simulink model "Ejercicio_Teorica_Simulink_1_MK2"  (R2024a)
settings: Solver=VariableStepAuto  StartTime=0.0  StopTime=20.0  RelTol=1e-3
undefined symbols (not defined in the file or in its folder): C, mat_K, mat_K_ampliada, mat_Ki, sustitu_mat_lin_A, sustitu_mat_lin_B
settings Model: Creator=juanj  LastModifiedBy=juanj
settings RTWCC: GPUComputeCapability=3.5

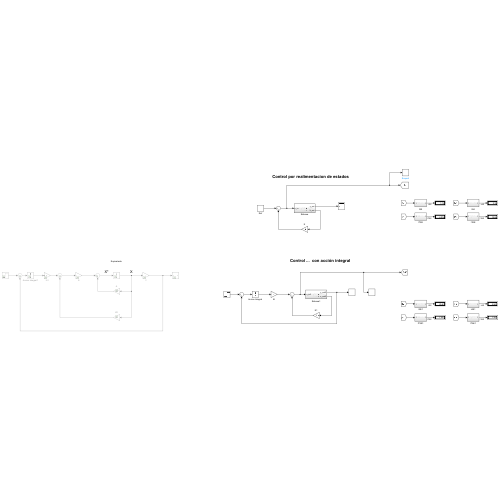
[thumbnail: Simulink's stored preview of the top-level diagram]
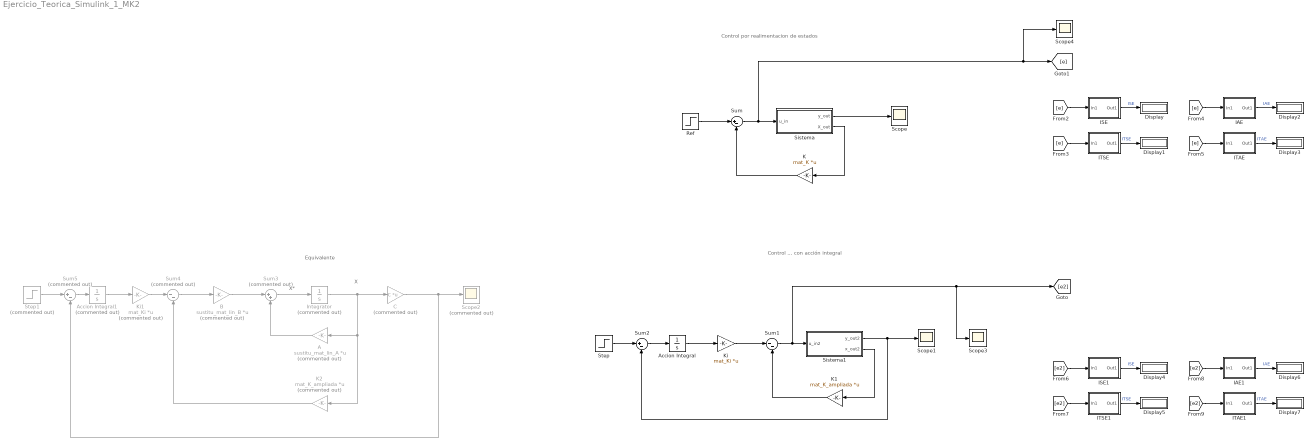
== system Ejercicio_Teorica_Simulink_1_MK2 ==
  note: Control ... con acción integral
  note: Equivalente
  note: X*
  note: X
  note: Control por realimentacion de estados
  A : Gain  Commented=on  Gain=sustitu_mat_lin_A  Multiplication=Matrix(K*u)
  Accion Integral : Integrator
  Accion Integral1 : Integrator  Commented=on
  B : Gain  Commented=on  Gain=sustitu_mat_lin_B  Multiplication=Matrix(K*u)
  C : Gain  Commented=on  Gain=C  Multiplication=Matrix(K*u)
  Display{,1..7} (8 alike) : Display
  IAE : Subsystem
  IAE1 : Subsystem
  ISE : Subsystem
  ISE1 : Subsystem
  ITAE : Subsystem
  ITAE1 : Subsystem
  ITSE : Subsystem
  ITSE1 : Subsystem
  Integrator : Integrator  Commented=on
  K : Gain  Gain=mat_K  Multiplication=Matrix(K*u)
  K1 : Gain  Gain=mat_K_ampliada  Multiplication=Matrix(K*u)
  K2 : Gain  Commented=on  Gain=mat_K_ampliada  Multiplication=Matrix(K*u)
  Ki : Gain  Gain=mat_Ki  Multiplication=Matrix(K*u)
  Ki1 : Gain  Commented=on  Gain=mat_Ki  Multiplication=Matrix(K*u)
  Ref : Step  Time=0  SampleTime=0
  Scope{,1,3..4} (4 alike) : Scope
  Scope2 : Scope  Commented=on
  Sistema : Subsystem
  Sistema1 : Subsystem
  Step : Step  Time=0  SampleTime=0
  Step1 : Step  Commented=on  Time=0  SampleTime=0
  Sum : Sum  Inputs=|+-
  Sum1 : Sum  Inputs=|--
  Sum2 : Sum  Inputs=|+-
  Sum3 : Sum  Commented=on  Inputs=|++
  Sum4 : Sum  Commented=on  Inputs=|--
  Sum5 : Sum  Commented=on  Inputs=|+-
  wires:
  Ref/1 -> Sum/1
  Sistema/1(y_out) -> Scope/1
  Sistema/2(X_out) -> K/1
  K/1 -> Sum/2
  Sistema1/1(y_out2) -> Scope1/1, Sum2/2
  Accion Integral/1 -> Ki/1
  Sum2/1 -> Accion Integral/1
  K1/1 -> Sum1/2
  Ki/1 -> Sum1/1
  Step/1 -> Sum2/1
  Sistema1/2(x_out2) -> K1/1
  Sum3/1 -> Integrator/1
  Sum4/1 -> B/1
  Integrator/1 -> K2/1, A/1, C/1
  A/1 -> Sum3/2
  B/1 -> Sum3/1
  K2/1 -> Sum4/2
  Ki1/1 -> Sum4/1
  Accion Integral1/1 -> Ki1/1
  Step1/1 -> Sum5/1
  Sum5/1 -> Accion Integral1/1
  C/1 -> Sum5/2, Scope2/1
  [e] -> ISE/1(In1)
  ISE/1(Out1) -> Display/1  "ISE"
  [e] -> ITAE/1(In1)
  ITSE/1(Out1) -> Display1/1  "ITSE"
  [e] -> ITSE/1(In1)
  ITAE/1(Out1) -> Display3/1  "ITAE"
  [e] -> IAE/1(In1)
  IAE/1(Out1) -> Display2/1  "IAE"
  [e2] -> ITAE1/1(In1)
  [e2] -> ISE1/1(In1)
  [e2] -> IAE1/1(In1)
  [e2] -> ITSE1/1(In1)
  ITAE1/1(Out1) -> Display7/1  "ITAE"
  IAE1/1(Out1) -> Display6/1  "IAE"
  ITSE1/1(Out1) -> Display5/1  "ITSE"
  ISE1/1(Out1) -> Display4/1  "ISE"
  Sum/1 -> Sistema/1(u_in), Scope4/1, [e]
  Sum1/1 -> [e2], Scope3/1, Sistema1/1(u_in2)

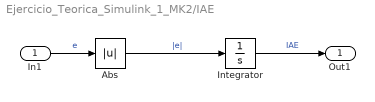
== system Ejercicio_Teorica_Simulink_1_MK2/IAE ==
  In1 : Inport
  Abs : Abs  SaturateOnIntegerOverflow=off
  Integrator : Integrator
  Out1 : Outport
  wires:
  Integrator/1 -> Out1/1  "IAE"
  In1/1 -> Abs/1  "e"
  Abs/1 -> Integrator/1  "|e|"

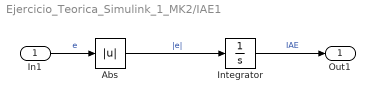
== system Ejercicio_Teorica_Simulink_1_MK2/IAE1 ==
  In1 : Inport
  Abs : Abs  SaturateOnIntegerOverflow=off
  Integrator : Integrator
  Out1 : Outport
  wires:
  Integrator/1 -> Out1/1  "IAE"
  In1/1 -> Abs/1  "e"
  Abs/1 -> Integrator/1  "|e|"

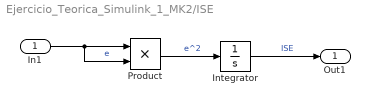
== system Ejercicio_Teorica_Simulink_1_MK2/ISE ==
  In1 : Inport
  Integrator : Integrator
  Product : Product
  Out1 : Outport
  wires:
  In1/1 -> Product/2, Product/1  "e"
  Product/1 -> Integrator/1  "e^2"
  Integrator/1 -> Out1/1  "ISE"

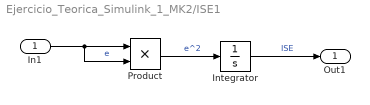
== system Ejercicio_Teorica_Simulink_1_MK2/ISE1 ==
  In1 : Inport
  Integrator : Integrator
  Product : Product
  Out1 : Outport
  wires:
  In1/1 -> Product/2, Product/1  "e"
  Product/1 -> Integrator/1  "e^2"
  Integrator/1 -> Out1/1  "ISE"

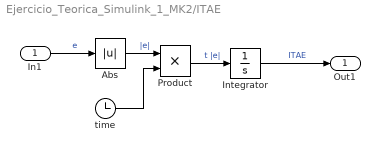
== system Ejercicio_Teorica_Simulink_1_MK2/ITAE ==
  In1 : Inport
  Abs : Abs  SaturateOnIntegerOverflow=off
  Integrator : Integrator
  Product : Product
  time : Clock
  Out1 : Outport
  wires:
  In1/1 -> Abs/1  "e"
  Integrator/1 -> Out1/1  "ITAE"
  time/1 -> Product/2
  Abs/1 -> Product/1  "|e|"
  Product/1 -> Integrator/1  "t |e|"

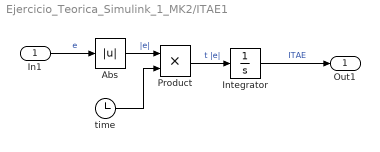
== system Ejercicio_Teorica_Simulink_1_MK2/ITAE1 ==
  In1 : Inport
  Abs : Abs  SaturateOnIntegerOverflow=off
  Integrator : Integrator
  Product : Product
  time : Clock
  Out1 : Outport
  wires:
  In1/1 -> Abs/1  "e"
  Integrator/1 -> Out1/1  "ITAE"
  time/1 -> Product/2
  Abs/1 -> Product/1  "|e|"
  Product/1 -> Integrator/1  "t |e|"

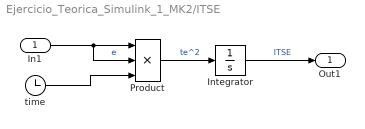
== system Ejercicio_Teorica_Simulink_1_MK2/ITSE ==
  In1 : Inport
  Integrator : Integrator
  Product : Product  Inputs=3
  time : Clock
  Out1 : Outport
  wires:
  Integrator/1 -> Out1/1  "ITSE"
  In1/1 -> Product/1, Product/2  "e"
  time/1 -> Product/3
  Product/1 -> Integrator/1  "te^2"

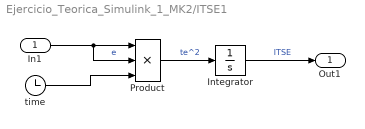
== system Ejercicio_Teorica_Simulink_1_MK2/ITSE1 ==
  In1 : Inport
  Integrator : Integrator
  Product : Product  Inputs=3
  time : Clock
  Out1 : Outport
  wires:
  Integrator/1 -> Out1/1  "ITSE"
  In1/1 -> Product/1, Product/2  "e"
  time/1 -> Product/3
  Product/1 -> Integrator/1  "te^2"

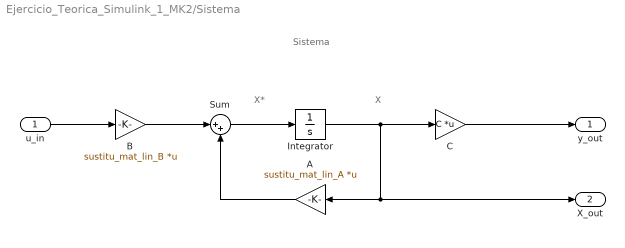
== system Ejercicio_Teorica_Simulink_1_MK2/Sistema ==
  note: Sistema
  note: X*
  note: X
  u_in : Inport
  A : Gain  Gain=sustitu_mat_lin_A  Multiplication=Matrix(K*u)
  B : Gain  Gain=sustitu_mat_lin_B  Multiplication=Matrix(K*u)
  C : Gain  Gain=C  Multiplication=Matrix(K*u)
  Integrator : Integrator
  Sum : Sum  Inputs=|++
  y_out : Outport
  X_out : Outport  Port=2
  wires:
  u_in/1 -> B/1
  A/1 -> Sum/2
  Sum/1 -> Integrator/1
  B/1 -> Sum/1
  Integrator/1 -> X_out/1, A/1, C/1
  C/1 -> y_out/1

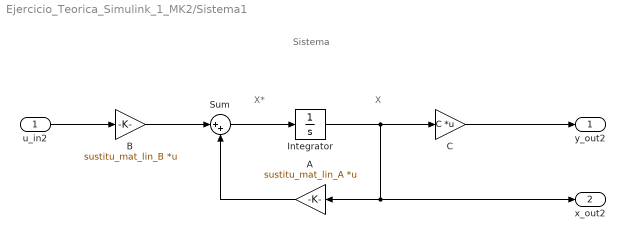
== system Ejercicio_Teorica_Simulink_1_MK2/Sistema1 ==
  note: Sistema
  note: X*
  note: X
  u_in2 : Inport
  A : Gain  Gain=sustitu_mat_lin_A  Multiplication=Matrix(K*u)
  B : Gain  Gain=sustitu_mat_lin_B  Multiplication=Matrix(K*u)
  C : Gain  Gain=C  Multiplication=Matrix(K*u)
  Integrator : Integrator
  Sum : Sum  Inputs=|++
  y_out2 : Outport
  x_out2 : Outport  Port=2
  wires:
  u_in2/1 -> B/1
  A/1 -> Sum/2
  Sum/1 -> Integrator/1
  C/1 -> y_out2/1
  B/1 -> Sum/1
  Integrator/1 -> x_out2/1, A/1, C/1
